simulink model "kukaslxctrlDemo"  (R2016a)
settings: Solver=ode5  StartTime=0.0  StopTime=inf  FixedStep=0.001  RelTol=1e-3
libraries: kukaslxctrl x2
settings Model: SimulationMode=external  Creator=julianleland  LastModifiedBy=julianleland
settings HardwareCC: ProdBitPerLong=64  ProdLargestAtomicFloat=None  ProdHWDeviceType=Intel->x86-64  TargetBitPerLong=64  TargetBitPerPointer=64  TargetIntDivRoundTo=Zero  TargetEndianess=LittleEndian  TargetWordSize=64  TargetHWDeviceType=Intel->x86-64
settings RTWCC: SystemTargetFile=sldrt.tlc  TemplateMakefile=sldrt.tmf  Description=Simulink Desktop Real-Time  RTWCompilerOptimization=on
settings CodeAppCC: MaxIdLength=95
settings SimulinkDesktopRealTimeCC: TargetPreCompLibLocation=/Applications/MATLAB_R2016a.app/toolbox/sldrt/lib/maci64  TargetLangStandard=C89/C90 (ANSI)  SupportVariableSizeSignals=off

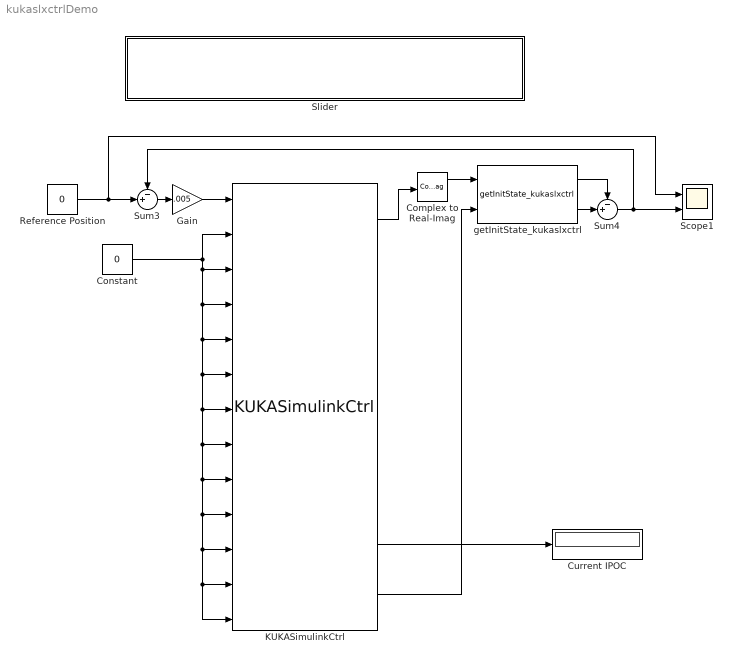
== system kukaslxctrlDemo ==
  Complex to Real-Imag : ComplexToRealImag
  Constant : Constant  Value=0
  Current IPOC : Display
  Gain : Gain  Gain=.005
  KUKASimulinkCtrl : kukaslxctrl/KUKASimulinkCtrl
  Reference Position : Constant  Value=0
  Scope1 : Scope  NumInputPorts=2
  Slider : Subsystem  DialogController=hmiCreateDDGDialog  IsWebBlock=on  mask(MWDashboardBlock){webBlockId=ecd4f56a-e48d-4b8a-89b0-8b23b0e88b89, webBlockType=slider, ShowInLibBrowser=on, ShowInitialText=on, HMISrcModelName=kukaslxctrlDemo}
      mask prompts: webBlockId "WebBlock Id"; webBlockType "WebBlock Type"; HMISrcModelName "Source Model"
      mask Help: helpview([docroot '/mapfiles/simulink.map'], 'hmi_slider')
      mask Display:
      | if strcmp(get_param(bdroot(gcb),'BlockDiagramType'), 'library')
      |     image([(matlabroot) '/toolbox/simulink/hmi/icons/Slider.png']);
      | end
  Sum3 : Sum  Inputs=-+|
  Sum4 : Sum  Inputs=-+|
  getInitState_kukaslxctrl : kukaslxctrl/getInitState_kukaslxctrl
  wires:
  Sum3/1 -> Gain/1
  Gain/1 -> KUKASimulinkCtrl/1
  Constant/1 -> KUKASimulinkCtrl/2, KUKASimulinkCtrl/3, KUKASimulinkCtrl/4, KUKASimulinkCtrl/5, KUKASimulinkCtrl/6, KUKASimulinkCtrl/7, KUKASimulinkCtrl/8, KUKASimulinkCtrl/9, KUKASimulinkCtrl/10, KUKASimulinkCtrl/11, KUKASimulinkCtrl/13, KUKASimulinkCtrl/12
  Sum4/1 -> Scope1/2, Sum3/1
  Reference Position/1 -> Scope1/1, Sum3/2
  KUKASimulinkCtrl/1 -> Complex to Real-Imag/1
  Complex to Real-Imag/1 -> getInitState_kukaslxctrl/1
  getInitState_kukaslxctrl/2 -> Sum4/2
  getInitState_kukaslxctrl/1 -> Sum4/1
  KUKASimulinkCtrl/16 -> getInitState_kukaslxctrl/2
  KUKASimulinkCtrl/14 -> Current IPOC/1

== system kukaslxctrlDemo/Slider ==
